simulink model "Lab_5_CAN_ECU2_1"  (R2014a)
settings: Solver=FixedStepDiscrete  StartTime=0.0  StopTime=10.0  RelTol=1e-3
undefined symbols (not defined in the file or in its folder): DEV, ECU565, motohawk_build_version, motohawk_trunc_name, motohawk_vardec_path, PROD
libraries: MotoHawk_lib x18, MotoHawk_Protocols_lib x1
settings Model: MotoHawkModelSavedName=Lab_5_CAN_ECU2_1  MotoHawkModelGUID=8BF714D2-C699-4C5B-8307-ED06704B45F6  MotoHawkModelOpenTime=2016 4 1 1 5 3.805  MotoHawkBuildVersion=035  MotoHawkBuildStats=struct('TotalFLASH',{0},'TotalEEPROM',{0},'TotalRAM',{0},'AppFLASH',{0},'AppEEPROM',{0},'AppRAM',{0},'HeapRAM',{0},'BuildSuccessCount',{35},'BuildErrorCount',{5})  MotoHawkBuildDirectory=C:\Users\Pradeep\Documents\MATLAB\DECS\Lab5\Lab5_03-09-2016\Lab5\Lab_5_CAN_ECU2_Build  MotoHawkBuildInfo=struct('model_name',{'Lab_5_CAN_ECU2'},'motohawk_version',{'2014a_sp3.1030'},'motohawk_component_version',{'0.0.8'},'matlab_version',{'8.3.0'},'build_version',{'034'},'module_type',{'ECU565-128'},'layout_type',{'DEV+PROD'},'processor_family',{'PPC'},'processor_type',{'MPC565'},'toolchain_vendor',{'gcc-powerpc-eabi'},'toolchain_version',{'4.6.0'},'component',{0},'archive_file',{'PCM128.a'},'enable_build',{1},'fptype',{0},'flash_size',{1048576},'ee_size',{8192},'ram_size',{36864},'decram_size',{4096},'eri_table0_rev',{9},'max_eri_table_size',{65535},'fgnd_base_period_ms',{5},'bgnd_base_period_ms',{50},'build_dir',{'H:\MATLAB\DECS\Lab5\Lab5\Lab_5_CAN_ECU2_Build'},'dll_name',{'Lab_5_CAN_034'},'srz_name',{'Lab_5_CAN_ECU2_034'},'fgnd_stack_size',{3072},'fgnd_angle_stack_size',{0},'bgnd_stack_size',{2048},'idle_stack_size',{1024},'irq_stack_size',{1536},'heap_size',{4096},'heap_margin',{409},'install_dll_dir',{'C:\ECUFiles\TDBDLL'},'install_srz_dir',{'C:\ECUFiles\Programs'},'app_int_stack_size',{1024},'shutdown_stack_size',{1024},'mingw_dir',{'C:\Program Files (x86)\Woodward\DevelopmentTools\Toolchains\GCC\win32-pe\4_7_0'},'motohawk_dir',{'C:\Program Files (x86)\Woodward\MCS\MotoHawk\2014a_sp3.1030'},'toolchain_dir',{'C:\Program Files (x86)\Woodward\DevelopmentTools\Toolchains\GCC\powerpc-eabi\4_6_0'},'matlab_root',{'C:\Program Files\MATLAB\2014a'},'model_guid',{'15C0F475-DB45-4760-96FC-AF2EF3AC3DC5'},'build_guid',{'8F91B811-C2FA-41C4-A125-45FA0F324F5E'},'token_guid',{'CAF9938D42F7BA4685752B9D7F66F53E'})  MotoHawkModelElapsedTime=251015.855  MotoHawkBuildGUID=8F91B811-C2FA-41C4-A125-45FA0F324F5E  CovSFcnEnable=on  Creator=hemant6043  LastModifiedBy=srini
settings ConfigSet: Description="This Simulink Configuration Set is preconfigured  for the MotoHawk target \"ECU565-128\"."
settings OptimizationCC: InlineParams=on  InlineInvariantSignals=on  EnhancedBackFolding=on  InitFltsAndDblsToZero=on  NoFixptDivByZeroProtection=on  EfficientFloat2IntCast=on  OptimizeModelRefInitCode=on  LifeSpan=1  SimCompilerOptimization=off
settings DebuggingCC: UnderspecifiedInitializationDetection=Classic  SolverPrmCheckMsg=none  InheritedTsInSrcMsg=none  TasksWithSamePriorityMsg=none  FrameProcessingCompatibilityMsg=error  ModelReferenceIOMismatchMessage=warning
settings HardwareCC: ProdLargestAtomicInteger=Integer  ProdLargestAtomicFloat=Float  ProdEndianess=BigEndian  ProdHWDeviceType=Specified
settings ModelReferenceCC: UpdateModelReferenceTargets=IfOutOfDate  CheckModelReferenceTargetMessage=warning  ModelReferenceNumInstancesAllowed=Single
settings RTWCC: SystemTargetFile=motohawk_ert_rtw.tlc  MakeCommand=make_rtw_motohawk  TemplateMakefile=motohawk_ert_rtw.tmf  Description=MotoHawk(tm) Rapid Prototyping  RTWCompilerOptimization=off
settings CodeAppCC: IgnoreCustomStorageClasses=off  MaxIdLength=100  CustomSymbolStrType=$N$R$M  CustomSymbolStrField=$H$N$M  InternalIdentifier=Classic
settings STFCustomTargetCC: ERTMultiwordTypeDef=User defined  ERTMultiwordLength=0  ConcurrentExecutionCompliant=off  IncludeMdlTerminateFcn=off  CombineOutputUpdateFcns=on  SuppressErrorStatus=on  ERTCustomFileBanners=on  SupportContinuousTime=off  SupportNonInlinedSFcns=off  MATLABClassNameForMDSCustomization=Simulink.SoftwareTarget.ERTCustomization  GRTInterface=off  SystemTargetFile=motohawk_ert_rtw.tlc
settings ERTTargetCC: ERTMultiwordTypeDef=User defined  ERTMultiwordLength=0  GenerateSampleERTMain=off  IncludeMdlTerminateFcn=off  GeneratePreprocessorConditionals=Disable all  SuppressErrorStatus=on  ERTCustomFileTemplate=motohawk_file_process.tlc

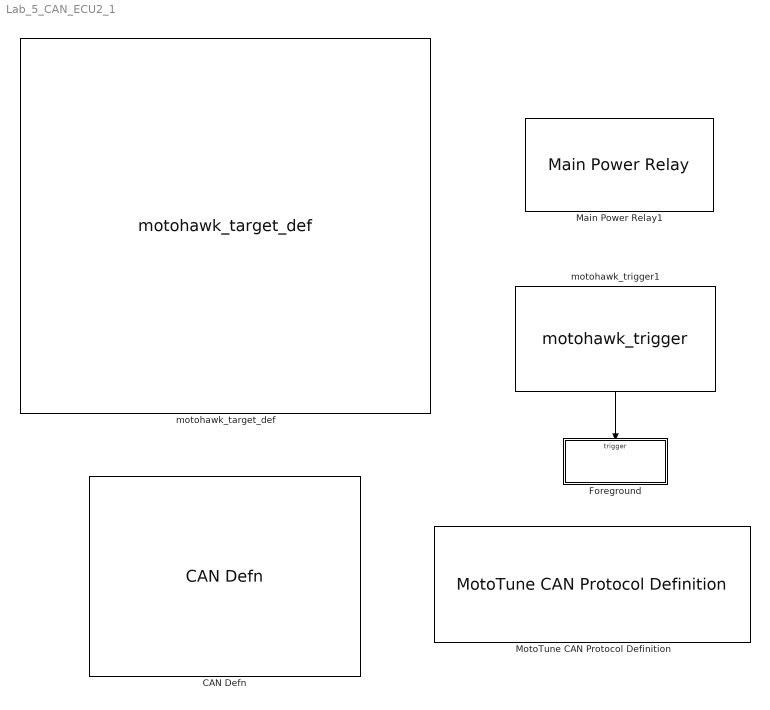
== system Lab_5_CAN_ECU2_1 ==
  CAN Defn : MotoHawk_lib/CAN Blocks/CAN Defn  Priority=-100  res_name='CAN_1'  text_resource=CAN1  target=ECU565-128  bit_time_src=Default  btime=250000  baud_rate_src=Constant  baud_rate=uint32(250000)  baud_rate_data_store_name='CAN1_BaudRate'  sample_point_tq_src=Constant  sample_point_tq=6  sample_point_tq_data_store_name='SamplePoint_TQ'  total_tq_src=Constant  total_tq=8  total_tq_data_store_name='Total_TQ'  synch_jw_src=Constant  synch_jw=1  synch_jw_data_store_name='SynchJumpWidth'  tx_queue_size=16  rx_queue_size=16
  Foreground : Subsystem  TreatAsAtomicUnit=on
  Main Power Relay1 : MotoHawk_lib/Extra Development Blocks/Main Power Relay  on_delay_count=2  off_delay_count=5  ecup_threshold=100  group='System | Main Power Relay'
  MotoTune CAN Protocol Definition : MotoHawk_Protocols_lib/MotoTune Blocks/MotoTune CAN Protocol Definition  Priority=-100  nam='MotoTuneHandler'  ref_name='CAN_1'  city_id_src=Constant  city_id=hex2dec('0C')  city_id_data_store_name='CityID'
  motohawk_target_def : MotoHawk_lib/motohawk_target_def  Priority=-65535  target=ECU565-128  layout=DEV+PROD  fptype=single (32 bits)  fgnd_stack_size=3*1024  fgnd_angle_stack_size=0  bgnd_stack_size=2*1024  idle_stack_size=1024  irq_stack_size=1536  app_int_stack_size=1024  shutdown_stack_size=1024  heap_size=4*1024  show_margins=off  fgnd_stack_margin=(3*1024) * 0.1  fgnd_angle_stack_margin=0  bgnd_stack_margin=(2*1024) * 0.1  idle_stack_margin=(1024) * 0.1  irq_stack_margin=(1536) * 0.1  app_int_stack_margin=(1024) * 0.1  shutdown_stack_margin=(1024) * 0.1  heap_margin=(4*1024) * 0.1  comp_name=bdroot  comp_img='KVASER_CAN_USB.jpg'  comp_security=No Encryption  comp_build_pass='mhbuild'  comp_sim_pass='mhsim'  comp_multi=off  show_filenames=off  dll_name=motohawk_trunc_name(bdroot, ['_' motohawk_build_version], 13)  srz_name=motohawk_trunc_name(bdroot, ['_' motohawk_build_version], 50)  build_dir='.'  comp_dir='.'
  motohawk_trigger1 : MotoHawk_lib/Trigger Blocks/motohawk_trigger  Tag=Trigger  Priority=0  trig_name=[]  trigger=FGND_RTI_PERIODIC  priority_order=0  inherited=off  run_disabled=off  override_app_monitor=off  target=ECU565_128
  wires:
  motohawk_trigger1/1 -> Foreground/Trigger

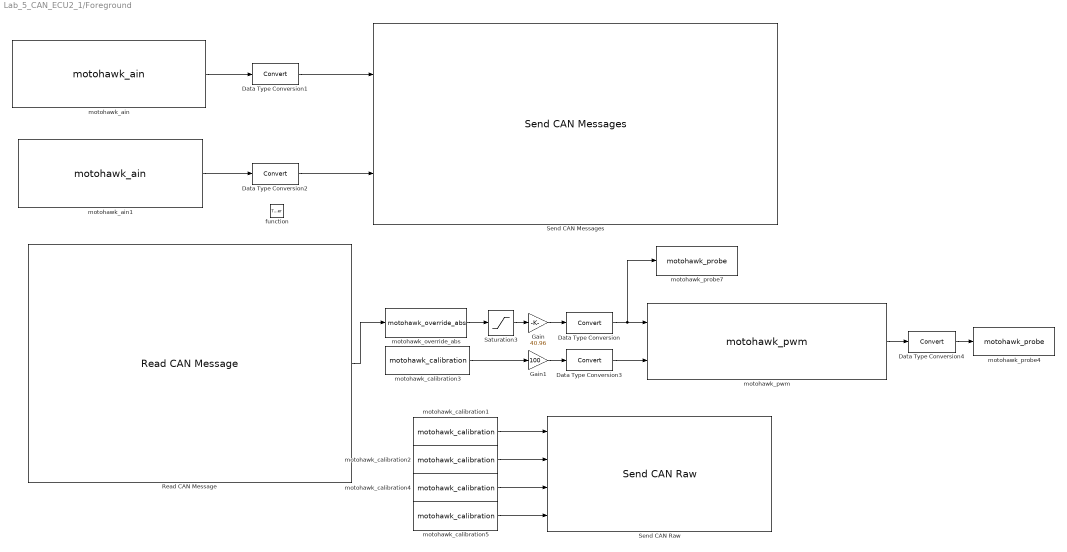
== system Lab_5_CAN_ECU2_1/Foreground ==
  function : TriggerPort  TriggerType=function-call
  Data Type Conversion{,1..4} (5 alike) : DataTypeConversion
  Gain : Gain  Gain=40.96
  Gain1 : Gain  Gain=100
  Read CAN Message : MotoHawk_lib/CAN Blocks/Read CAN Message  nam='CAN_1'  bus=-2  msg=etc_can_600  queue=1  slot=''  valid=off  stale=off  labelwires=off
  Saturation3 : Saturate  UpperLimit=80  LowerLimit=-80
  Send CAN Messages : MotoHawk_lib/CAN Blocks/Send CAN Messages  bus=-2  nam='CAN_1'  msgl=etc_can_500  pace=5  labelwires=off
  Send CAN Raw : MotoHawk_lib/CAN Blocks/Send CAN Raw  nam='CAN_1'  bus=-2  interval=10
  motohawk_ain : MotoHawk_lib/Analog I//O Blocks/motohawk_ain  res_name=[]  text_resource=AN5M  code_resource=NONE  val_resource=-1  target=ECU565-128  resource_enum_str=(None)=-1,ECUP=53,DRVP=54,XDRP=55,AN1M=56,AN2M=57,AN3M=58,AN4M=59,AN5M=60,AN6M=61,AN7M=62,AN8M=63,AN9M=64,AN10M=65,AN11M=66,AN12M=67,AN13M=68,AN14M=69,AN15M=70,AN16M=71,AN17M=72,AN18M=73,AN19M=74,AN20M=75,AN21M=76,AN22M=77,AN23M=78,AN24M=79,AN25M=80,AN26M=81,AN27M=82,AN28M=83,AN29M=84,AN30M=85,AN31M=86,AN32M=87,AN33M=88,AN34M=89,O2A=90,O2B=91,XDRP_B=92,REF_14V=143  altref=5V Reference  typ=uint16  num_adc_bits=10  use_stat=off  use_vardec=off  nam='RTD1_MW'  read_level=1  write_level=1  group='System | I/O Pins | Inputs Config'
  motohawk_ain1 : MotoHawk_lib/Analog I//O Blocks/motohawk_ain  res_name=[]  text_resource=AN4M  code_resource=NONE  val_resource=-1  target=ECU565-128  resource_enum_str=(None)=-1,ECUP=53,DRVP=54,XDRP=55,AN1M=56,AN2M=57,AN3M=58,AN4M=59,AN5M=60,AN6M=61,AN7M=62,AN8M=63,AN9M=64,AN10M=65,AN11M=66,AN12M=67,AN13M=68,AN14M=69,AN15M=70,AN16M=71,AN17M=72,AN18M=73,AN19M=74,AN20M=75,AN21M=76,AN22M=77,AN23M=78,AN24M=79,AN25M=80,AN26M=81,AN27M=82,AN28M=83,AN29M=84,AN30M=85,AN31M=86,AN32M=87,AN33M=88,AN34M=89,O2A=90,O2B=91,XDRP_B=92,REF_14V=143  altref=5V Reference  typ=uint16  num_adc_bits=10  use_stat=off  use_vardec=off  nam='RTD1_MW'  read_level=1  write_level=1  group='System | I/O Pins | Inputs Config'
  motohawk_calibration1 : MotoHawk_lib/Calibration & Probing Blocks/motohawk_calibration  nam='IDType'  val=0  storage=Display  show_more=off  name_source=Use Parameter  data_type=Inherit from 'Default Value'  read_level=1  write_level=1  ovr_cals=on  view_as=Number  enum_struct={'Disabled', 'Enabled'}  vector_style=Wide Row  use_help_units=off  help=''  units=''  use_header_enum=off  row_header_enum={}  col_header_enum={}  use_min_max=off  min_val=-inf  max_val=inf  use_precision=off  precision=''  gain=1  offset=0  exp=1  use_mototune_group=off  mototune_group=motohawk_vardec_path(gcb)  data_stores=motohawk_sfun_calibration_data_stores
  motohawk_calibration2 : MotoHawk_lib/Calibration & Probing Blocks/motohawk_calibration  nam='ID'  val=1024  storage=Display  show_more=off  name_source=Use Parameter  data_type=Inherit from 'Default Value'  read_level=1  write_level=1  ovr_cals=on  view_as=Number  enum_struct={'Disabled', 'Enabled'}  vector_style=Wide Row  use_help_units=off  help=''  units=''  use_header_enum=off  row_header_enum={}  col_header_enum={}  use_min_max=off  min_val=-inf  max_val=inf  use_precision=off  precision=''  gain=1  offset=0  exp=1  use_mototune_group=off  mototune_group=motohawk_vardec_path(gcb)  data_stores=motohawk_sfun_calibration_data_stores
  motohawk_calibration3 : MotoHawk_lib/Calibration & Probing Blocks/motohawk_calibration  nam='ETC_freq'  val=5000  storage=Calibration  show_more=off  name_source=Use Parameter  data_type=Inherit from 'Default Value'  read_level=1  write_level=1  ovr_cals=on  view_as=Number  enum_struct={'Disabled', 'Enabled'}  vector_style=Wide Row  use_help_units=off  help=''  units=''  use_header_enum=off  row_header_enum={}  col_header_enum={}  use_min_max=off  min_val=-inf  max_val=inf  use_precision=off  precision=''  gain=1  offset=0  exp=1  use_mototune_group=off  mototune_group=motohawk_vardec_path(gcb)  data_stores=motohawk_sfun_calibration_data_stores
  motohawk_calibration4 : MotoHawk_lib/Calibration & Probing Blocks/motohawk_calibration  nam='DataLength'  val=0  storage=Display  show_more=off  name_source=Use Parameter  data_type=Inherit from 'Default Value'  read_level=1  write_level=1  ovr_cals=on  view_as=Number  enum_struct={'Disabled', 'Enabled'}  vector_style=Wide Row  use_help_units=off  help=''  units=''  use_header_enum=off  row_header_enum={}  col_header_enum={}  use_min_max=off  min_val=-inf  max_val=inf  use_precision=off  precision=''  gain=1  offset=0  exp=1  use_mototune_group=off  mototune_group=motohawk_vardec_path(gcb)  data_stores=motohawk_sfun_calibration_data_stores
  motohawk_calibration5 : MotoHawk_lib/Calibration & Probing Blocks/motohawk_calibration  nam='Data'  val=[0 0 0 0 0 0 0 0]  storage=Display  show_more=off  name_source=Use Parameter  data_type=Inherit from 'Default Value'  read_level=1  write_level=1  ovr_cals=on  view_as=Number  enum_struct={'Disabled', 'Enabled'}  vector_style=Wide Row  use_help_units=off  help=''  units=''  use_header_enum=off  row_header_enum={}  col_header_enum={}  use_min_max=off  min_val=-inf  max_val=inf  use_precision=off  precision=''  gain=1  offset=0  exp=1  use_mototune_group=off  mototune_group=motohawk_vardec_path(gcb)  data_stores=motohawk_sfun_calibration_data_stores
  motohawk_override_abs : MotoHawk_lib/Calibration & Probing Blocks/motohawk_override_abs  parent_name='ETC_Duty_Cycle'  parent_val=0  show_more=off  name_source=Use Parameter  parent_read_level=1  parent_override_level=1  view_as=Number  enum_struct={'Disabled', 'Enabled'}  use_help_units=off  parent_help=''  parent_units=''  use_min_max=off  parent_min=-inf  parent_max=inf  use_precision=off  parent_precision=''  parent_gain=1  parent_offset=0  parent_exp=1  use_mototune_group=off  parent_group=motohawk_vardec_path(gcb)
  motohawk_probe4 : MotoHawk_lib/Calibration & Probing Blocks/motohawk_probe  nam='HBridge_current'  show_more=off  name_source=Use Parameter  read_level=1  view_as=Number  enum_struct={'Disabled', 'Enabled'}  vector_style=Wide Row  use_help_units=off  help=''  units=''  use_header_enum=off  row_header_enum={}  col_header_enum={}  use_min_max=off  min_val=-inf  max_val=inf  use_precision=off  precision=''  gain=1  offset=0  exp=1  use_mototune_group=off  mototune_group=motohawk_vardec_path(gcb)
  motohawk_probe7 : MotoHawk_lib/Calibration & Probing Blocks/motohawk_probe  nam='Dutycyle'  show_more=off  name_source=Use Parameter  read_level=1  view_as=Number  enum_struct={'Disabled', 'Enabled'}  vector_style=Wide Row  use_help_units=off  help=''  units=''  use_header_enum=off  row_header_enum={}  col_header_enum={}  use_min_max=off  min_val=-inf  max_val=inf  use_precision=off  precision=''  gain=1  offset=0  exp=1  use_mototune_group=off  mototune_group=motohawk_vardec_path(gcb)
  motohawk_pwm : MotoHawk_lib/Analog I//O Blocks/motohawk_pwm  res_name=[]  text_resource=H1  target=ECU565-128  freq_mode=-1  min_freq=5000  use_max_freq=off  max_freq=20000  use_enable=off  use_brake=off  output_current=on  output_fault_status=off  use_child=off  use_vardec=off  nam='PWMOutput'  read_level=1  write_level=1  group='System | I/O Pins | Outputs Config'
  wires:
  motohawk_ain/1 -> Data Type Conversion1/1
  motohawk_ain1/1 -> Data Type Conversion2/1
  motohawk_pwm/1 -> Data Type Conversion4/1
  motohawk_calibration3/1 -> Gain1/1
  Gain/1 -> Data Type Conversion/1
  Data Type Conversion/1 -> motohawk_probe7/1, motohawk_pwm/1
  Data Type Conversion3/1 -> motohawk_pwm/2
  Gain1/1 -> Data Type Conversion3/1
  Data Type Conversion4/1 -> motohawk_probe4/1
  motohawk_override_abs/1 -> Saturation3/1
  Saturation3/1 -> Gain/1
  Read CAN Message/1 -> motohawk_override_abs/1
  Data Type Conversion1/1 -> Send CAN Messages/1
  Data Type Conversion2/1 -> Send CAN Messages/2
  motohawk_calibration1/1 -> Send CAN Raw/1
  motohawk_calibration2/1 -> Send CAN Raw/2
  motohawk_calibration4/1 -> Send CAN Raw/3
  motohawk_calibration5/1 -> Send CAN Raw/4
